simulink model "sf_msg_process_multiple_messages"  (R2017b)
settings: Solver=VariableStepAuto  StartTime=0.0  StopTime=10.0  RelTol=1e-3  EnableMultiTasking=on
settings Model: Creator=The MathWorks, Inc.  LastModifiedBy=The MathWorks, Inc.
settings DataIOCC: LimitDataPoints=on
settings OptimizationCC: LifeSpan=inf
settings DebuggingCC: AllowSymbolicDim=off  SFUnexpectedBacktrackingDiag=warning  SFNoUnconditionalDefaultTransitionDiag=warning  SFExecutionAtInitializationDiag=none
settings ModelReferenceCC: PropagateSignalLabelsOutOfModel=off
settings CodeAppCC: StateflowObjectComments=on
settings GRTTargetCC: TargetLangStandard=C89/C90 (ANSI)
settings ConfigComp: CovMetricSettings=dw  CovHtmlReporting=on  CovSaveCumulativeToWorkspaceVar=on  CovSaveSingleToWorkspaceVar=on  CovExternalEMLEnable=off

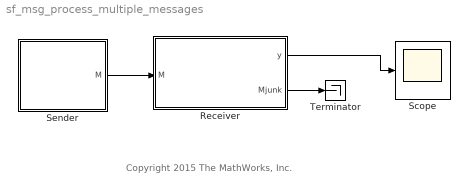
== system sf_msg_process_multiple_messages ==
  note: Copyright 2015 The MathWorks, Inc.
  Receiver : Stateflow chart  TreatAsAtomicUnit=on
  Scope : Scope
  Sender : Stateflow chart  TreatAsAtomicUnit=on
  Terminator : Terminator
  wires:
  Sender/1(M) -> Receiver/1(M)
  Receiver/1(y) -> Scope/1
  Receiver/2(Mjunk) -> Terminator/1

== stateflow chart sf_msg_process_multiple_messages/Receiver ==
  state Init
  state yy = sumOfAllMessageData [function]
    (default) -> (junction 15) : {yy = 0;}
    (junction 15) -> (junction 14) [order 1] : M
    (junction 14) -> (junction 16) : {
        | yy = yy + M.data;
        | forward(M, Mjunk);
        | }
    (junction 16) -> (junction 15)
    (junction 15) -> (junction 17) [order 2]
  state ProcessAllMessages
    en:
    y = sumOfAllMessageData();
  (default) -> Init
  Init -> ProcessAllMessages : after(5,sec)
  data: yy function_output; y output; M input; Mjunk output =0

== stateflow chart sf_msg_process_multiple_messages/Sender ==
  state A
    en:
    M.data = 1;
    send(M);
    M.data = 2;
    send(M);
    M.data = 3;
    send(M);
  data: M output
